simulink model "Seguidordelinea"  (R2015a)
settings: Solver=ode45  StartTime=0.0  StopTime=inf  RelTol=1e-3
libraries: fuzblock x1, instrumentlib x1
settings Model: Creator=Asus  LastModifiedBy=Asus

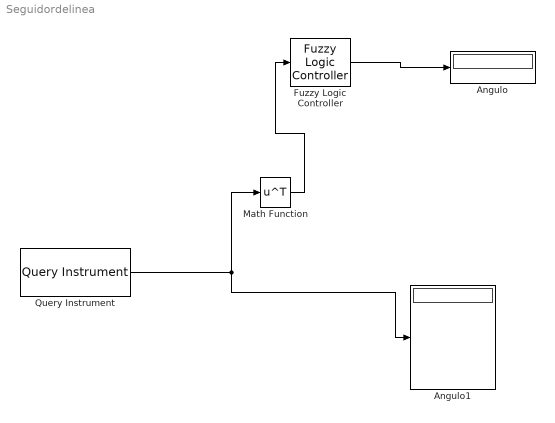
== system Seguidordelinea ==
  Angulo : Display
  Angulo1 : Display
  Fuzzy Logic Controller : fuzblock/Fuzzy Logic  Controller  fis='seguirlinea.fis'
  Math Function : Math  Operator=transpose  OutMin=[5]  OutMax=[5]  SaturateOnIntegerOverflow=on
  Query Instrument : instrumentlib/Query Instrument  sampleTime=1  isWorkspaceObject=off  timeout=10  inputBufferSize=512  protocol=Serial  serialPort=COM3  baudRate=9600  gpibVendor=Advantech  boardIndex=0  primaryAddress=1  secondaryAddress=0  visaVendor=Agilent  visaSerialPort=0  chassisIndex=0  logicalAddress=0  tcpRemoteHost='127.0.0.1'  tcpRemotePort=4500  udpRemoteHost='127.0.0.1'  udpRemotePort=9090  visaTCPBoardIndex=0  visaTCPRemoteHost='127.0.0.1'  usbBoardIndex=0  usbManufID=0  usbModelCode=0  usbSerialNumber=0  initAction=None  initCommand='DATA:SOURCE CH1'  initFunction=get  queryCommand='curve?'  responseFormat=ASCII  asciiFormatting='%d'  precision=8-bit integer  byteOrder=Little Endian  valuesToRead=1  removeBytes=off  afterOutputAction=Repeat query for new data  enableFrames=on  frameSize=5
  wires:
  Fuzzy Logic Controller/1 -> Angulo/1
  Query Instrument/1 -> Angulo1/1, Math Function/1
  Math Function/1 -> Fuzzy Logic Controller/1
